simulink model "rc_response"  (R2024a)
settings: Solver=VariableStepAuto  StartTime=0.0  StopTime=51  RelTol=1e-3
undefined symbols (not defined in the file): LF
libraries: instrumentseriallib x3
settings Model: Creator=osoko  LastModifiedBy=osoko

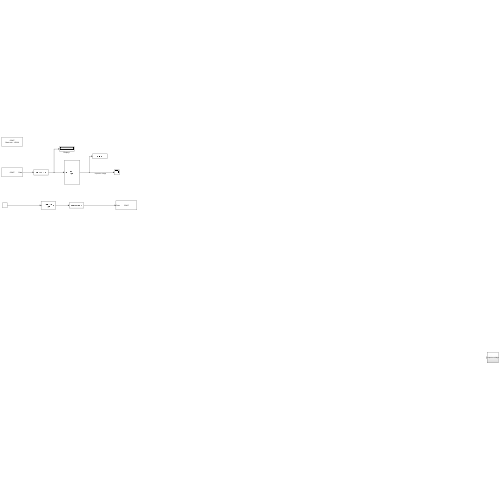
[thumbnail: Simulink's stored preview of the top-level diagram]
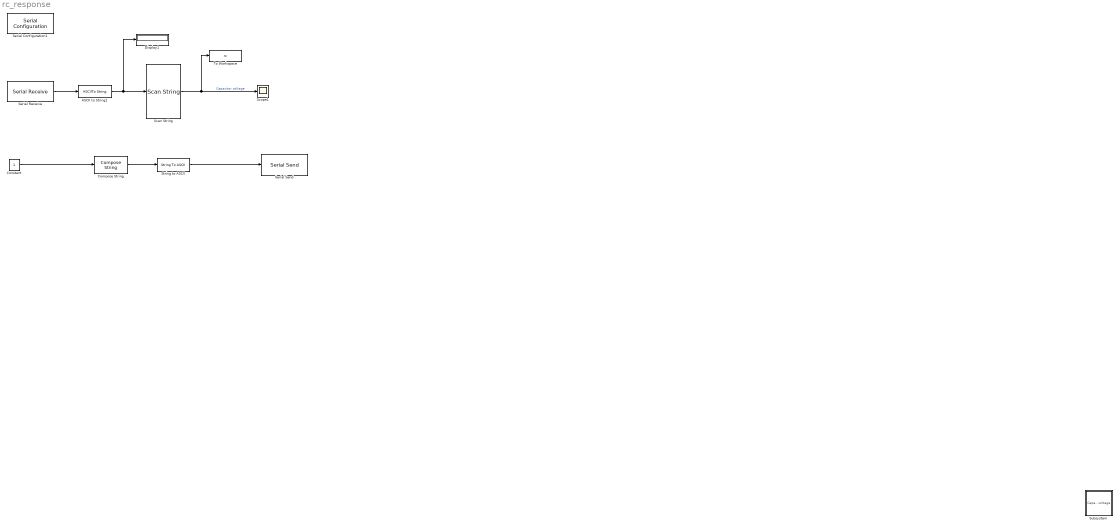
== system rc_response ==
  ASCII to String1 : ASCIIToString
  Compose String : ComposeString  Format="\"V,%f\""
  Constant : Constant
  Display1 : Display
      settings: Decimation=3
  Scan String : ScanString  Format="\"%f\""
  Scope1 : Scope
  Serial Configuration1 : instrumentseriallib/Serial Configuration  Priority=-200000  PortSel=COM7  Port=COM7  ComPort=COM7  BaudRate=115200  DataBits=8  Parity=none  StopBits=1  ByteOrder=little-endian  FlowControl=none  Timeout=10  SimulateUsing=Interpreted execution  BlockInModel=on  aMode=1
  Serial Receive : instrumentseriallib/Serial Receive  Priority=1  PortSel=COM7  Port=COM7  ComPort=COM7  DataType=uint8  SaveDataType=uint8  ToggleHeader=off  Header=[]  ToggleDataSize=on  DataSize=[5]  ToggleTerminator=on  Terminator=LF ('\n')  CustomTerminator=[]  InputFormat=Column major  EnableBlockingMode=on  ActionDataUnavailable=Output last received value  ActionWhenDataUnavailable=Output last received value  CustomValue=0  SampleTime=0.01  SimulateUsing=Interpreted execution  BlockInModel=on  aMode=1
  Serial Send : instrumentseriallib/Serial Send  Priority=1  PortSel=COM7  Port=COM7  ComPort=COM7  Header=[]  Terminator=LF ('\n')  CustomTerminator=[]  EnableBlockingMode=on  SimulateUsing=Interpreted execution  BlockInModel=on  aMode=1
  String to ASCII : StringToASCII
  Subsystem : Subsystem
  To Workspace : ToWorkspace  VariableName=rc  SaveFormat=Timeseries  SampleTime=-1
  wires:
  Serial Receive/1 -> ASCII to String1/1
  ASCII to String1/1 -> Display1/1, Scan String/1
  Scan String/1 -> To Workspace/1, Scope1/1  "Capacitor voltage"
  Compose String/1 -> String to ASCII/1
  Constant/1 -> Compose String/1
  String to ASCII/1 -> Serial Send/1

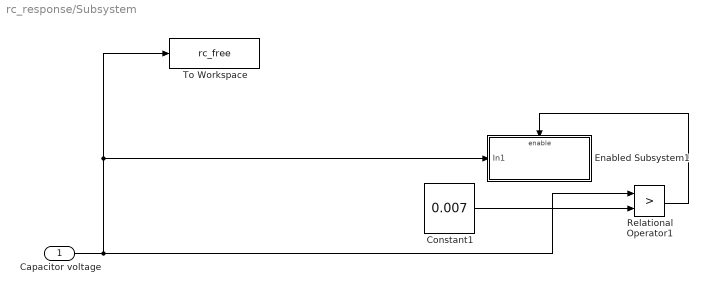
== system rc_response/Subsystem ==
  Capacitor voltage : Inport
  Constant1 : Constant  Value=0.007  VectorParams1D=off  SampleTime=-1
  Enabled Subsystem1 : Subsystem  TreatAsAtomicUnit=on
  Relational Operator1 : RelationalOperator  Operator=>  OutDataTypeStr=boolean  RndMeth=Simplest  InputSameDT=off
  To Workspace : ToWorkspace  VariableName=rc_free  SaveFormat=Structure With Time  SampleTime=-1
  wires:
  Relational Operator1/1 -> Enabled Subsystem1/Enable
  Constant1/1 -> Relational Operator1/2
  Capacitor voltage/1 -> To Workspace/1, Enabled Subsystem1/1(In1), Relational Operator1/1

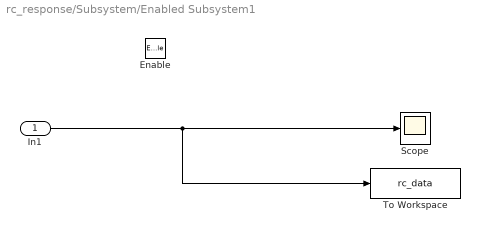
== system rc_response/Subsystem/Enabled Subsystem1 ==
  In1 : Inport
  Enable : EnablePort
  Scope : Scope
  To Workspace : ToWorkspace  VariableName=rc_data  SaveFormat=Structure With Time  SampleTime=-1
  wires:
  In1/1 -> Scope/1, To Workspace/1
